simulink model "UAVbackstepping"  (Simulink 10.3)
settings: Solver=FixedStepAuto  StartTime=0.0  StopTime=100  FixedStep=0.01  RelTol=1e-3  EnableMultiTasking=on
settings Model: LogicAnalyzerSignalOrdering=b46eab1f-6d7b-46d5-ba77-869c9bcf8073,e372ee43-6b29-46b4-abe2-21db8a75f3db,54536452-6e4b-4c4e-8d4d-0328bb149ba5,ee120f98-b3af-4c2b-98e6-fd07fbf403a8,95f0ccf8-e806-4aca-b244-47a68f5b17c2,43173032-e17e-41b3-ae27-c107c89a8554,cd05f008-1193-4f09-83b2-320887a6bfed,77335dc1-2049-4d60-adff-c5cf65fb9f9c,2b0633ed-ee51-4564-bd40-7c1ecd56d7dd,dfe04f60-c018-4575-84ca-0f2bc48ccfdd,15828245-0370-4267-bd56-27ac584a7d3e,a94eabd6-13e1-4944-88ab-4db36129ad16,2589506c-7c8c-49ed-89a6-d105e2fe226b,cee16f5b-ea6a-452d-9ab2-cf488d9efbab,cfbac93e-1ce9-416b-a9d8-bf10efdf7acc,4b85f622-f658-405c-8f3b-f9afb204eecf,74d215f9-d3fc-487f-9be0-003869bd056c,b88364f3-47d2-4798-9ca3-2210a76b2151,992ed9bb-61c6-4816-9df8-a6a9b01ec379,fa3f50c4-9508-49a0-8b01-2ac87a115d50,443bea33-00d3-41d7-a326-92ebc5658bd2,b9b4d7ee-6fc8-43e3-85dd-aee403bc8ecc,493d881f-12cd-495e-8dbc-5128311b9c68,b5f602f6-6904-40bd-b13c-e30cee082fb3,ac9778e8-5991-4c7f-a0e3-96968d354415,7bf7420a-51df-410a-ad7d-640b8e127968,6783366a-253d-440d-8309-d3e37f712b7a,e3002545-8a11-46c6-8ec8-6cad10b13a30,8d9e8d02-f9c8-417c-9dde-eafb8a0edd13,386452ee-c7b4-48c3-9b3b-9b5c8c01b9d9,a3f579f7-78fa-4a39-bc72-402bae468470,1b92f911-6c45-4a57-9771-5ef78c83ee6e,46570d27-1e42-4fbc-a47b-5b7b35a38f8f,e5c679aa-f5c2-4db1-b0e0-4143dc9292e5,653c2844-e192-4241-9d80-46dbab4f59eb,a81b4801-5ad4-47ee-be3a-7b6b03c586a0,9c2d5a89-a715-4e09-b03f-f97d33dae6e2,bbe3c297-77a7-404c-8c78-a013d080af9d,25508a3f-0527-4920-9e54-841bdeffa537,04472a12-bcc6-4a52-8174-bab8d6a6428e,43579eec-1d9f-48b6-9500-b23169589754,13906945-f0a2-42b5-a059-d3263a4d8fea,5debfe0f-7549-4053-9490-66e9123c9aa5,ba1e7171-ac89-4725-b702-5e8a13beef21,88975c86-fcb6-4eb7-a3b3-cfbaa1f90a45,5938fb88-f0d0-465a-95d6-16780bbd5b65,12608a54-9dd1-42f3-95f2-303540ea6fbd,e0fdc368-fa77-4673-aa31-0c283bfe0d72,9baec6ec-eb92-460d-8517-da3730d3c5a9,b421fcc5-0c1c-4c89-ba38-a7c1f88a7f58,8eabe517-0bde-4a7e-9911-b56cb8fb40be,d2f80fa9-708b-426c-89bf-a5279d614744,4ff3bab7-3c7f-4ac4-b9a7-239084307073,16cb91f4-d8fb-4662-979f-86f54ca22852,694bc1bc-d9f8-4696-9709-c2a3c0b4c400,9b3c29cc-2abe-4d54-a9dd-6ec7aa243ded,9a8a996a-a39e-40af-b6f5-e33e96ef8062,4edc1bd5-7ef1-4e99-9f98-7b7c38d83df9,574ec7e1-1a45-4502-b5ca-a33a3001e453,54705b3a-a62a-42de-9894-18fee6dd9f2f,52cc81ea-ec29-4b3c-a7fa-d0b8a74c3977,40c87669-2e0a-4c05-aa3c-23dbde47ecaf,8d820c60-f138-442a-a396-16a173d0311b,099a5a67-d92d-4072-ac0a-dca54051a8b8,37013ffe-99d3-4146-a42e-9df11827c8f0  Creator=Administrator  LastModifiedBy=duolan  MultithreadedSim=on
settings DataIOCC: LimitDataPoints=on  SignalLoggingSaveFormat=Dataset
settings OptimizationCC: ExpressionDepthLimit=128
settings DebuggingCC: UnderspecifiedInitializationDetection=Simplified  MergeDetectMultiDrivingBlocksExec=error  SolverPrmCheckMsg=warning  FcnCallInpInsideContextMsg=error  StateNameClashWarn=none
settings GRTTargetCC: CombineOutputUpdateFcns=on  GRTInterface=off
settings ConfigComp: CovSFcnEnable=off

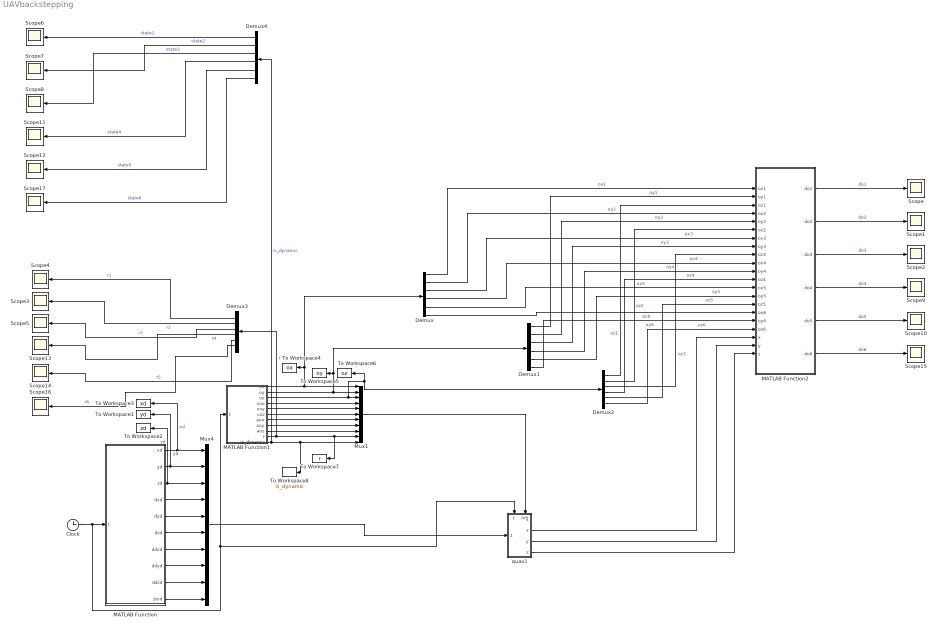
== system UAVbackstepping ==
  Clock : Clock
  Demux{,1..4} (5 alike) : Demux  Outputs=6
  MATLAB Function : MATLAB Function  TreatAsAtomicUnit=on
  MATLAB Function1 : MATLAB Function  TreatAsAtomicUnit=on
  MATLAB Function2 : MATLAB Function  TreatAsAtomicUnit=on
  Mux1 : Mux  Inputs=11
  Mux4 : Mux  Inputs=10
  Scope{,1..17} (18 alike) : Scope
  To Workspace1 : ToWorkspace  VariableName=yd  SampleTime=-1
  To Workspace2 : ToWorkspace  VariableName=zd  SampleTime=-1
  To Workspace3 : ToWorkspace  VariableName=xd  SampleTime=-1
  To Workspace4 : ToWorkspace  VariableName=ox  SampleTime=-1
  To Workspace5 : ToWorkspace  VariableName=oy  SampleTime=-1
  To Workspace6 : ToWorkspace  VariableName=oz  SampleTime=-1
  To Workspace7 : ToWorkspace  VariableName=r  SampleTime=-1
  To Workspace8 : ToWorkspace  VariableName=is_dynamic  SampleTime=-1
  quav1 : Subsystem
      settings: PortSchema="{\"entries\":[{\"content\":{\"sides\":[{\"content\":{\"connectorIds\":[\"In1\"]},\"type\":\"ConnectorPlacement.EquallySpacedRectSide\",\"uuid\":\"dcfd3588-1954-4120-b512-4285ff7746bb\"},{\"content\":{\"connectorIds\":[\"Out1\",\"Out2\",\"Out3\",\"Out4\"],\"side\":\"RIGHT\"},\"type\":\"ConnectorPlacement.EquallySpacedRectSide\",\"uuid\":\"6db42291-2fd7-4549-90c1-3af3d88c1f44\"},{\"content\":{\"connectorIds\":[\"In2\",\"In3\"],\"side\":\"TOP\"},\"type\":\"ConnectorPlacement.EquallySpacedRectSide\",\"uuid\":\"9b3b6533-6a28-4d06-948b-5572cd3b642f\"}]},\"type\":\"ConnectorPlacement.EquallySpacedConnector\",\"uuid\":\"66a38cae-fd35-47b9-aceb-4f0f598ddd12\"}],\"packageUris\":[\"http://schema.mathworks.com/mf0/Connector/R2020b\"],\"version\":\"1.0\"}"
  wires:
  MATLAB Function/2(yd) -> To Workspace1/1, Mux4/2  "yd"
  MATLAB Function/3(zd) -> Mux4/3, To Workspace2/1  "zd"
  MATLAB Function/1(xd) -> To Workspace3/1, Mux4/1  "xd"
  MATLAB Function/4(dxd) -> Mux4/4
  MATLAB Function/5(dyd) -> Mux4/5
  MATLAB Function/6(dzd) -> Mux4/6
  MATLAB Function/7(ddxd) -> Mux4/7
  MATLAB Function/8(ddyd) -> Mux4/8
  MATLAB Function/9(ddzd) -> Mux4/9
  MATLAB Function/10(psid) -> Mux4/10
  Mux4/1 -> quav1/1(In1)
  Clock/1 -> quav1/2(t), MATLAB Function1/1(t), MATLAB Function/1(t)
  MATLAB Function1/1(ox) -> Mux1/1, Demux/1, To Workspace4/1
  MATLAB Function1/2(oy) -> Mux1/2, Demux1/1, To Workspace5/1
  MATLAB Function1/3(oz) -> Mux1/3, To Workspace6/1, Demux2/1
  Mux1/1 -> quav1/3(In5)
  MATLAB Function1/4(vox) -> Mux1/4
  MATLAB Function1/5(voy) -> Mux1/5
  MATLAB Function1/6(voz) -> Mux1/6
  MATLAB Function1/7(aox) -> Mux1/7
  MATLAB Function1/8(aoy) -> Mux1/8
  MATLAB Function1/9(aoz) -> Mux1/9
  MATLAB Function1/10(r) -> Demux3/1, To Workspace7/1, Mux1/10  "r"
  MATLAB Function1/11(is_dynamic) -> To Workspace8/1, Mux1/11, Demux4/1  "is_dynamic"
  MATLAB Function2/1(do1) -> Scope/1  "do1"
  MATLAB Function2/2(do2) -> Scope1/1  "do2"
  MATLAB Function2/3(do3) -> Scope2/1  "do3"
  quav1/2(x) -> MATLAB Function2/19(x)
  quav1/3(y) -> MATLAB Function2/20(y)
  quav1/4(z) -> MATLAB Function2/21(z)
  Demux3/1 -> Scope4/1  "r1"
  Demux3/2 -> Scope3/1  "r2"
  Demux3/3 -> Scope5/1  "r3"
  Demux4/1 -> Scope6/1  "state1"
  Demux4/2 -> Scope7/1  "state2"
  Demux4/3 -> Scope8/1  "state3"
  Demux/1 -> MATLAB Function2/1(ox1)  "ox1"
  Demux1/1 -> MATLAB Function2/2(oy1)  "oy1"
  Demux2/1 -> MATLAB Function2/3(oz1)  "oz1"
  Demux/2 -> MATLAB Function2/4(ox2)  "ox2"
  Demux1/2 -> MATLAB Function2/5(oy2)  "oy2"
  Demux2/2 -> MATLAB Function2/6(oz2)  "oz2"
  Demux/3 -> MATLAB Function2/7(ox3)  "ox3"
  Demux1/3 -> MATLAB Function2/8(oy3)  "oy3"
  Demux2/3 -> MATLAB Function2/9(oz3)  "oz3"
  Demux/4 -> MATLAB Function2/10(ox4)  "ox4"
  Demux1/4 -> MATLAB Function2/11(oy4)  "oy4"
  Demux/5 -> MATLAB Function2/13(ox5)  "ox5"
  Demux1/5 -> MATLAB Function2/14(oy5)  "oy5"
  Demux2/5 -> MATLAB Function2/15(oz5)  "oz5"
  MATLAB Function2/4(do4) -> Scope9/1  "do4"
  MATLAB Function2/5(do5) -> Scope10/1  "do5"
  Demux2/4 -> MATLAB Function2/12(oz4)  "oz4"
  Demux4/4 -> Scope11/1  "state4"
  Demux4/5 -> Scope12/1  "state5"
  Demux3/4 -> Scope13/1  "r4"
  Demux3/5 -> Scope14/1  "r5"
  Demux/6 -> MATLAB Function2/16(ox6)  "ox6"
  Demux1/6 -> MATLAB Function2/17(oy6)  "oy6"
  Demux2/6 -> MATLAB Function2/18(oz6)  "oz6"
  MATLAB Function2/6(do6) -> Scope15/1  "do6"
  Demux3/6 -> Scope16/1  "r6"
  Demux4/6 -> Scope17/1  "state6"

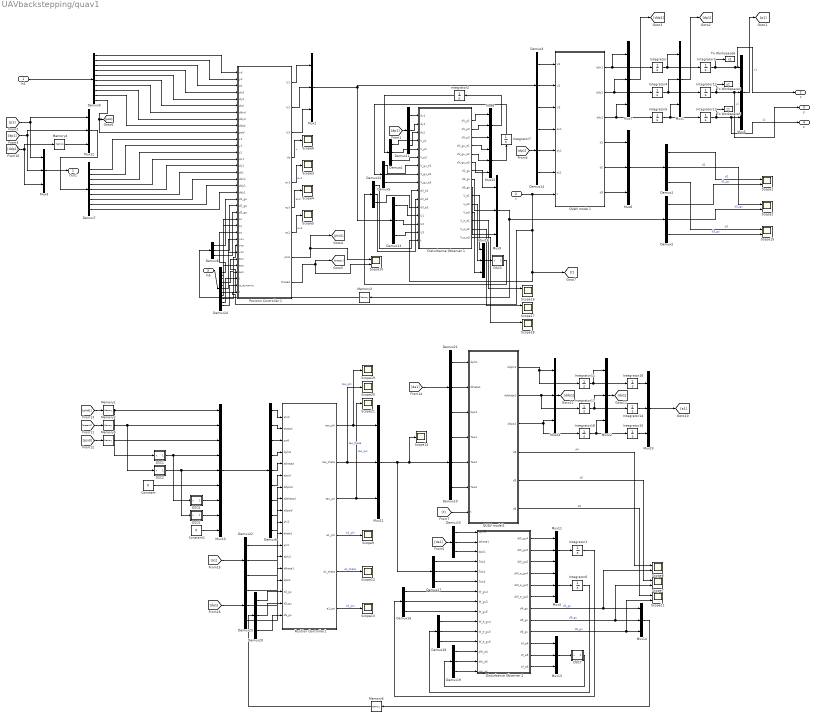
== system UAVbackstepping/quav1 ==
  In1 : Inport
  t : Inport  Port=2
  In5 : Inport  Port=3
  Constant : Constant  Value=0
  Constant1 : Constant  Value=0
  DSC1 : Subsystem
  DSC2 : Subsystem
  DSC3 : Subsystem
  DSC4 : Subsystem
  DSC5 : Subsystem
  DSC7 : Subsystem
  Demux{1..5,8,10..23} (20 alike) : Demux  Outputs=3
  Demux24 : Demux  Outputs=11
  Demux6 : Demux  Outputs=9
  Demux7 : Demux  Outputs=9
  Demux9 : Demux  Outputs=10
  Disturbance Observer 1 : MATLAB Function  TreatAsAtomicUnit=on
  Disturbance Observer 2 : MATLAB Function  TreatAsAtomicUnit=on
  Integrator{,1..2,4..7,11..18} (15 alike) : Integrator
  Integrator3 : Integrator  InitialCondition=1
  Memory{1..4,6} (5 alike) : Memory
  Memory5 : Memory  InitialCondition=pi/3
  Mux{1..9,11..16,21..24} (19 alike) : Mux  Inputs=3
  Mux10 : Mux  Inputs=9
  Position Controller 1 : MATLAB Function  TreatAsAtomicUnit=on
  Position Controller1 : MATLAB Function  TreatAsAtomicUnit=on
  QUAV mode 1 : MATLAB Function  TreatAsAtomicUnit=on
  QUAV model1 : MATLAB Function  TreatAsAtomicUnit=on
  Scope{1..2,7..8,10..11,15..18} (10 alike) : Scope  NumInputPorts=2
  Scope{3..6,9,12..14,19..21} (11 alike) : Scope
  To Workspace4 : ToWorkspace  VariableName=y1  SampleTime=-1
  To Workspace5 : ToWorkspace  VariableName=z1  SampleTime=-1
  To Workspace6 : ToWorkspace  VariableName=x1  SampleTime=-1
  Out1 : Outport
  x : Outport  Port=2
  y : Outport  Port=3
  z : Outport  Port=4
  wires:
  Demux7/5 -> Position Controller 1/15(dy1)
  Position Controller 1/2(U2) -> Mux1/2
  QUAV mode 1/1(ddx1) -> Mux7/1, Integrator/1
  QUAV mode 1/3(ddz1) -> Mux7/3, Integrator5/1
  Disturbance Observer 1/2(dV_p2) -> Mux8/2
  Demux7/7 -> Position Controller 1/17(ddx1)
  Demux8/2 -> Position Controller 1/21(d2_gu)
  Integrator13/1 -> z/1, Mux5/3, To Workspace5/1  "z1"
  Demux7/3 -> Position Controller 1/13(z1)
  Disturbance Observer 1/9(d3_gu) -> Mux9/3
  Demux11/1 -> Disturbance Observer 1/1(dx1)
  Demux9/8 -> Position Controller 1/8(ddyd)
  Integrator4/1 -> Mux2/2, Integrator12/1
  Mux1/1 -> Demux3/1, Demux13/1
  Demux7/6 -> Position Controller 1/16(dz1)
  Demux9/3 -> Position Controller 1/3(zd)
  Demux9/10 -> [psid], Position Controller 1/10(psid)
  QUAV mode 1/5(d2) -> Mux6/2
  [dp1] -> Demux14/1
  Memory3/1 -> Demux8/1
  Demux3/3 -> QUAV mode 1/3(U3)
  Mux2/1 -> [dp1]
  Demux7/8 -> Position Controller 1/18(ddy1)
  Demux3/2 -> QUAV mode 1/2(U2)
  Demux7/9 -> Position Controller 1/19(ddz1)
  Demux14/3 -> QUAV mode 1/6(dz1)
  QUAV mode 1/2(ddy1) -> Mux7/2, Integrator4/1
  Demux9/6 -> Position Controller 1/6(dzd)
  Demux14/2 -> QUAV mode 1/5(dy1)
  [ddp1] -> Mux3/3, Memory4/1
  Position Controller 1/1(U1) -> Mux1/1
  Demux9/7 -> Position Controller 1/7(ddxd)
  Integrator5/1 -> Mux2/3, Integrator13/1
  Integrator/1 -> Mux2/1, Integrator3/1
  Demux3/1 -> QUAV mode 1/1(U1)
  QUAV mode 1/6(d3) -> Mux6/3
  Demux9/4 -> Position Controller 1/4(dxd)
  Position Controller 1/4(Up) -> Scope6/1  "u"
  Memory4/1 -> Mux12/3
  Demux13/1 -> Disturbance Observer 1/13(U1)
  Demux7/4 -> Position Controller 1/14(dx1)
  Demux11/2 -> Disturbance Observer 1/2(dy1)
  Mux6/1 -> Demux1/1
  Mux5/1 -> [p1]
  Demux13/3 -> Disturbance Observer 1/15(U3)
  Disturbance Observer 1/7(d1_gu) -> Mux9/1
  Disturbance Observer 1/8(d2_gu) -> Mux9/2
  Demux14/1 -> QUAV mode 1/4(dx1)
  Mux7/1 -> [ddp1]
  QUAV mode 1/4(d1) -> Mux6/1
  Demux11/3 -> Disturbance Observer 1/3(dz1)
  Position Controller 1/3(U3) -> Mux1/3
  Demux7/1 -> Position Controller 1/11(x1)
  Disturbance Observer 1/3(dV_p3) -> Mux8/3
  [dp1] -> Demux11/1
  Position Controller 1/6(ey1) -> Scope4/1  "ex2"
  Demux7/2 -> Position Controller 1/12(y1)
  Demux13/2 -> Disturbance Observer 1/14(U2)
  Disturbance Observer 1/1(dV_p1) -> Mux8/1
  Mux12/1 -> Demux7/1
  Position Controller 1/5(ex1) -> Scope3/1  "ex1"
  Integrator3/1 -> x/1, Mux5/1, To Workspace6/1  "x1"
  Demux8/3 -> Position Controller 1/22(d3_gu)
  Demux9/5 -> Position Controller 1/5(dyd)
  [dp1] -> Mux3/2, Mux12/2
  Position Controller 1/7(ez1) -> Scope5/1  "ex3"
  [p1] -> Mux3/1, Mux12/1
  Demux9/1 -> Position Controller 1/1(xd)
  Demux8/1 -> Position Controller 1/20(d1_gu)
  Demux9/2 -> Position Controller 1/2(yd)
  Demux9/9 -> Position Controller 1/9(ddzd)
  Integrator12/1 -> y/1, Mux5/2, To Workspace4/1  "y1"
  Mux9/1 -> Memory3/1, Demux2/1
  Mux8/1 -> Integrator2/1
  In1/1 -> Demux9/1
  Mux3/1 -> Out1/1
  t/1 -> Position Controller 1/34(t), Disturbance Observer 1/16(t), [t], QUAV mode 1/7(t)
  Position Controller 1/8(phid) -> [phid1], Scope10/1
  Position Controller 1/9(thetad) -> Scope10/2, [thetad1]
  QUAV model1/1(ddphi1) -> Integrator11/1, Mux24/1
  Mux22/1 -> [da1]
  Mux23/1 -> [a1]
  Demux6/7 -> Position Controller1/7(ddphid)
  Integrator14/1 -> Mux23/2
  [phid1] -> Memory1/1
  Demux23/1 -> Position Controller1/13(dphi1)
  Demux6/5 -> Position Controller1/5(dthetad)
  Position Controller1/6(e1_psi) -> Scope13/1  "e1_psi"
  Constant/1 -> Mux10/6
  Position Controller1/1(tao_phi) -> Scope19/1, Mux21/1  "tao_phi"
  Demux22/1 -> Position Controller1/10(phi1)
  Demux22/2 -> Position Controller1/11(theta1)
  DSC5/1(dx) -> Mux10/8
  Demux23/3 -> Position Controller1/15(dpsi1)
  Demux10/2 -> QUAV model1/5(Tao2)
  Demux6/8 -> Position Controller1/8(ddthetad)
  [thetad1] -> Memory2/1
  Position Controller1/4(e1_phi) -> Scope9/1  "e1_phi"
  Position Controller1/5(e1_theta) -> Scope12/1  "e1_theta"
  Demux10/1 -> QUAV model1/4(Tao1)
  [psid] -> Memory5/1
  Demux21/3 -> QUAV model1/3(dpsi1)
  DSC1/1(dx) -> DSC4/1(x), Mux10/4
  Demux21/1 -> QUAV model1/1(dphi1)
  Constant1/1 -> Mux10/9
  [da1] -> Demux23/1
  Demux21/2 -> QUAV model1/2(dtheta1)
  Demux23/2 -> Position Controller1/14(dtheta1)
  [da1] -> Demux21/1
  Integrator15/1 -> Mux23/3
  DSC2/1(dx) -> DSC5/1(x), Mux10/5
  Integrator18/1 -> Mux22/3, Integrator15/1
  QUAV model1/3(ddpsi1) -> Integrator18/1, Mux24/3
  Demux6/4 -> Position Controller1/4(dphid)
  Integrator11/1 -> Mux22/1, Integrator16/1
  Integrator17/1 -> Mux22/2, Integrator14/1
  Integrator16/1 -> Mux23/1
  Position Controller1/2(tao_theta) -> Scope20/1, Mux21/2  "tao_theta"
  Demux6/6 -> Position Controller1/6(dpsid)
  Position Controller1/3(tao_psi) -> Scope21/1, Mux21/3  "tao_psi"
  Mux10/1 -> Demux6/1
  [a1] -> Demux22/1
  Demux22/3 -> Position Controller1/12(psi1)
  Demux10/3 -> QUAV model1/6(Tao3)
  Demux6/9 -> Position Controller1/9(ddpsid)
  QUAV model1/2(ddtheta1) -> Integrator17/1, Mux24/2
  Mux21/1 -> Demux17/1, Scope14/1, Demux10/1
  Demux6/1 -> Position Controller1/1(phid)
  Demux6/3 -> Position Controller1/3(psid)
  DSC4/1(dx) -> Mux10/7
  Mux24/1 -> [dda1]
  Demux6/2 -> Position Controller1/2(thetad)
  Demux15/1 -> Disturbance Observer 2/1(dphi1)
  Demux15/2 -> Disturbance Observer 2/2(dtheta1)
  Demux15/3 -> Disturbance Observer 2/3(dpsi1)
  Disturbance Observer 2/1(dW_gu4) -> Mux11/1
  Disturbance Observer 2/2(dW_gu5) -> Mux11/2
  Disturbance Observer 2/3(dW_gu6) -> Mux11/3
  Mux11/1 -> Integrator1/1
  [da1] -> Demux15/1
  [t] -> QUAV model1/7(t)
  QUAV model1/4(d4) -> Scope8/1  "d4"
  QUAV model1/5(d5) -> Scope7/1  "d5"
  QUAV model1/6(d6) -> Scope11/1  "d6"
  Demux16/1 -> Disturbance Observer 2/7(W_gu4)
  Demux16/2 -> Disturbance Observer 2/8(W_gu5)
  Demux16/3 -> Disturbance Observer 2/9(W_gu6)
  Integrator1/1 -> Demux16/1
  Demux17/1 -> Disturbance Observer 2/4(Tao1)
  Demux17/2 -> Disturbance Observer 2/5(Tao2)
  Demux17/3 -> Disturbance Observer 2/6(Tao3)
  Disturbance Observer 2/7(d4_gu) -> Mux14/1, Scope8/2  "d4_gu"
  Disturbance Observer 2/8(d5_gu) -> Mux14/2, Scope7/2  "d5_gu"
  Disturbance Observer 2/9(d6_gu) -> Mux14/3, Scope11/2  "d6_gu"
  Disturbance Observer 2/5(dW_e_gu5) -> Mux4/2
  Disturbance Observer 2/4(dW_e_gu4) -> Mux4/1
  Mux4/1 -> Integrator6/1
  Disturbance Observer 2/6(dW_e_gu6) -> Mux4/3
  Demux18/1 -> Disturbance Observer 2/10(W_e_gu4)
  Demux18/2 -> Disturbance Observer 2/11(W_e_gu5)
  Demux18/3 -> Disturbance Observer 2/12(W_e_gu6)
  Integrator6/1 -> Demux18/1
  Disturbance Observer 2/10(W_e4) -> Mux13/1
  Disturbance Observer 2/11(W_e5) -> Mux13/2
  Disturbance Observer 2/12(W_e6) -> Mux13/3
  Mux13/1 -> DSC7/1(x)
  Demux19/1 -> Disturbance Observer 2/13(dW_e4)
  Demux19/2 -> Disturbance Observer 2/14(dW_e5)
  Demux19/3 -> Disturbance Observer 2/15(dW_e6)
  DSC7/1(dx) -> Demux19/1
  Mux14/1 -> Memory6/1
  Demux20/1 -> Position Controller1/16(d4_gu)
  Demux20/2 -> Position Controller1/17(d5_gu)
  Demux20/3 -> Position Controller1/18(d6_gu)
  Memory6/1 -> Demux20/1
  Memory1/1 -> DSC1/1(x), Mux10/1
  Memory2/1 -> DSC2/1(x), Mux10/2
  Memory5/1 -> Mux10/3
  In5/1 -> Demux24/1
  Demux24/1 -> Position Controller 1/23(ox)
  Demux24/2 -> Position Controller 1/24(oy)
  Demux24/3 -> Position Controller 1/25(oz)
  Demux24/4 -> Position Controller 1/26(vox)
  Demux24/5 -> Position Controller 1/27(voy)
  Demux24/6 -> Position Controller 1/28(voz)
  Demux24/7 -> Position Controller 1/29(aox)
  Demux24/8 -> Position Controller 1/30(aoy)
  Demux24/9 -> Position Controller 1/31(aoz)
  Demux24/10 -> Position Controller 1/32(r)
  Demux24/11 -> Position Controller 1/33(is_dynamic)
  Integrator2/1 -> Demux4/1
  Demux4/1 -> Disturbance Observer 1/4(V_p1)
  Demux4/2 -> Disturbance Observer 1/5(V_p2)
  Demux4/3 -> Disturbance Observer 1/6(V_p3)
  Disturbance Observer 1/4(dV_gu_e1) -> Mux15/1
  Disturbance Observer 1/5(dV_gu_e2) -> Mux15/2
  Disturbance Observer 1/6(dV_gu_e3) -> Mux15/3
  Mux15/1 -> Integrator7/1
  Integrator7/1 -> Demux5/1
  Demux5/1 -> Disturbance Observer 1/7(V_gu_e1)
  Demux5/2 -> Disturbance Observer 1/8(V_gu_e2)
  Demux5/3 -> Disturbance Observer 1/9(V_gu_e3)
  Disturbance Observer 1/10(V_e1) -> Mux16/1
  Disturbance Observer 1/11(V_e2) -> Mux16/2
  Disturbance Observer 1/12(V_e3) -> Mux16/3
  Mux16/1 -> DSC3/1(x)
  DSC3/1(dx) -> Demux12/1
  Demux12/1 -> Disturbance Observer 1/10(dV_e1)
  Demux12/2 -> Disturbance Observer 1/11(dV_e2)
  Demux12/3 -> Disturbance Observer 1/12(dV_e3)
  Demux1/1 -> Scope1/1  "d1"
  Demux2/1 -> Scope1/2  "d1_gu"
  Demux1/2 -> Scope2/1  "d2"
  Demux2/2 -> Scope2/2  "d2_gu"
  Demux1/3 -> Scope15/1  "d3"
  Demux2/3 -> Scope15/2  "d3_gu"
  Disturbance Observer 1/13(V_e_e1) -> Scope16/1
  Disturbance Observer 1/14(V_e_e2) -> Scope17/1
  Disturbance Observer 1/15(V_e_e3) -> Scope18/1

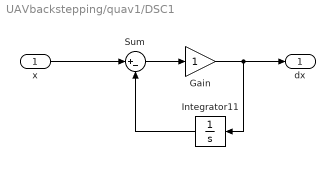
== system UAVbackstepping/quav1/DSC1 ==
  x : Inport
  Gain : Gain
  Integrator11 : Integrator
  Sum : Sum  Inputs=|+-
  dx : Outport
  wires:
  Sum/1 -> Gain/1
  x/1 -> Sum/1
  Integrator11/1 -> Sum/2
  Gain/1 -> Integrator11/1, dx/1

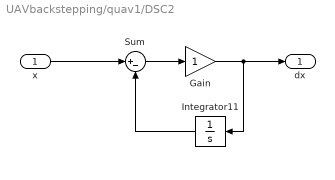
== system UAVbackstepping/quav1/DSC2 ==
  x : Inport
  Gain : Gain
  Integrator11 : Integrator
  Sum : Sum  Inputs=|+-
  dx : Outport
  wires:
  Sum/1 -> Gain/1
  x/1 -> Sum/1
  Integrator11/1 -> Sum/2
  Gain/1 -> Integrator11/1, dx/1

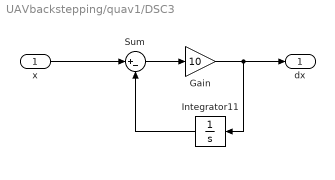
== system UAVbackstepping/quav1/DSC3 ==
  x : Inport
  Gain : Gain  Gain=10
  Integrator11 : Integrator
  Sum : Sum  Inputs=|+-
  dx : Outport
  wires:
  Sum/1 -> Gain/1
  x/1 -> Sum/1
  Integrator11/1 -> Sum/2
  Gain/1 -> Integrator11/1, dx/1

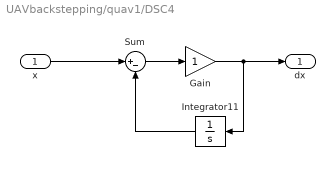
== system UAVbackstepping/quav1/DSC4 ==
  x : Inport
  Gain : Gain
  Integrator11 : Integrator
  Sum : Sum  Inputs=|+-
  dx : Outport
  wires:
  Sum/1 -> Gain/1
  x/1 -> Sum/1
  Integrator11/1 -> Sum/2
  Gain/1 -> Integrator11/1, dx/1

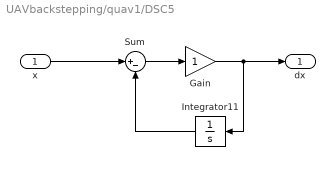
== system UAVbackstepping/quav1/DSC5 ==
  x : Inport
  Gain : Gain
  Integrator11 : Integrator
  Sum : Sum  Inputs=|+-
  dx : Outport
  wires:
  Sum/1 -> Gain/1
  x/1 -> Sum/1
  Integrator11/1 -> Sum/2
  Gain/1 -> Integrator11/1, dx/1

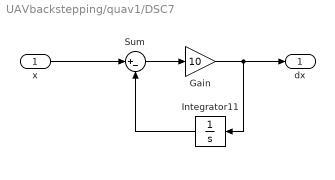
== system UAVbackstepping/quav1/DSC7 ==
  x : Inport
  Gain : Gain  Gain=10
  Integrator11 : Integrator
  Sum : Sum  Inputs=|+-
  dx : Outport
  wires:
  Sum/1 -> Gain/1
  x/1 -> Sum/1
  Integrator11/1 -> Sum/2
  Gain/1 -> Integrator11/1, dx/1

== matlab function quav1/Position Controller 1 ==
  data: xd input double; U1 output double; yd input double; zd input double; dxd input double; dyd input double; dzd input double; ddxd input double; ddyd input double; ddzd input double; psid input double; x1 input double; y1 input double; z1 input double; dx1 input double; dy1 input double; dz1 input double; ddx1 input double; ddy1 input double; ddz1 input double; U2 output double; U3 output double; Up output double; ex1 output double; ey1 output double; ez1 output double; d1_gu input double; d2_gu input double; d3_gu input double; phid output double; thetad output double; ox input double; oy input double; oz input double; vox input double; voy input double; voz input double; aox input double; aoy input double; aoz input double; r input double; is_dynamic input double; t input double
function [U1,U2,U3,Up,ex1,ey1,ez1,phid,thetad] = fcn(xd,yd,zd,dxd,dyd,dzd,ddxd,ddyd,ddzd,psid,x1,y1,z1,dx1,dy1,dz1,ddx1,ddy1,ddz1,d1_gu,d2_gu,d3_gu,ox,oy,oz,vox,voy,voz,aox,aoy,aoz,r,is_dynamic,t)

%postion parameter
K1=0.1;
K2=0.1;
K3=0.1;
m=2;
g=9.81;
es=0.01;


% error
ex1=x1-xd;
dex1=dx1-dxd;
ey1=y1-yd;
dey1=dy1-dyd;
ez1=z1-zd;
dez1=dz1-dzd;


% nominal control
es=0.01;
kex11=0.65;kex12=7/9;kex13=(2-kex12)*es^(kex12-1);kex14=(kex12-1)*es^(kex12-2);b1=0.65;
key11=0.5;key12=7/9;key13=(2-key12)*es^(key12-1);key14=(key12-1)*es^(key12-2);b2=0.5;
kez11=2.5;kez12=7/9;kez13=(2-kez12)*es^(kez12-1);kez14=(kez12-1)*es^(kez12-2);b3=2.5;

if abs(ex1)>es
    Lx1=kex11*((abs(ex1))^kex12)*sign(ex1);
else
    Lx1=kex13*ex1+kex14*ex1*ex1*sign(ex1);
end
if abs(ey1)>es
    Ly1=key11*((abs(ey1))^key12)*sign(ey1);
else
    Ly1=key13*ey1+key14*ey1*ey1*sign(ey1);
end
if abs(ez1)>es
    Lz1=kez11*((abs(ez1))^(kez12))*sign(ez1);
else
    Lz1=kez13*ez1+key14*ez1*ez1*sign(ez1);
end
sx1=dex1+b1*ex1+Lx1;
sy1=dey1+b2*ey1+Ly1;
sz1=dez1+b3*ez1+Lz1;

if abs(ex1)>es
    dLx1=kex11*kex12*((abs(ex1))^(kex12-1))*dex1;
else 
    dLx1=kex13*dex1+2*kex14*ex1*dex1*sign(ex1);
end
if abs(ey1)>es
    dLy1=key11*key12*((abs(ey1))^(key12-1))*dey1;
else
    dLy1=key13*dey1+2*key14*ey1*dey1*sign(ey1);
end
if abs(ez1)>es
    dLz1=kez11*kez12*((abs(ez1))^(kez12-1))*dez1;
else
    dLz1=kez13*dez1+2*kez14*ez1*dez1*sign(ez1);
end

U1=K1*dx1/m-d1_gu+ddxd-b1*dex1-dLx1-5*sx1-5*((abs(sx1))^(5/7))*sign(sx1);
U2=K2*dy1/m-d2_gu+ddyd-b2*dey1-dLy1-1.5*sy1-1.5*((abs(sy1))^(5/7))*sign(sy1);
U3=K3*dz1/m-d3_gu+g+ddzd-b3*dez1-dLz1-1.5*sz1-1.5*((abs(sz1))^(5/7))*sign(sz1);




%control barrier function
k1 = 4; k2 = 4;

num_obs = length(ox);  
A = zeros(num_obs, 3); 
b = zeros(num_obs, 1);

for i = 1:num_obs
    oxi = ox(i);
    oyi = oy(i);
    ozi = oz(i);
    voxi = vox(i);
    voyi = voy(i);
    vozi = voz(i);
    aoxi = aox(i);
    aoyi = aoy(i);
    aozi = aoz(i);
    ri  = r(i);
    
    % 
    h = (x1 - oxi)^2 + (y1 - oyi)^2 + (z1 - ozi)^2 - (ri+0.2)^2;
    dh = 2*(x1 - oxi)*(-voxi)+2*(x1 - oxi)*dx1 +2*(y1 - oyi)*(-voyi)+ 2*(y1 - oyi)*dy1 + 2*(z1 - ozi)*(-vozi)+2*(z1 - ozi)*dz1;
    dh1=2*(x1 - oxi)*dx1+ 2*(y1 - oyi)*dy1+2*(z1 - ozi)*dz1;
    % 
    A(i, :) = [-2*(x1 - oxi), -2*(y1 - oyi), -2*(z1 - ozi)];


    b(i) = 2*(x1 - oxi)*(-K1*dx1/m+d1_gu )-abs(2*(x1 - oxi))*2.5+ 2*(dx1^2)+2*(voxi^2)-4*voxi*dx1-2*(x1 - oxi)*aoxi+ ...
           2*(y1 - oyi)*(-K2*dy1/m+d2_gu )+ 2*(dy1^2)+2*(voyi^2)-4*voyi*dy1-2*(y1 - oyi)*aoyi +...
           2*(z1 - ozi)*(-K3*dz1/m - g+d3_gu)+ 2*(dz1^2)+2*(vozi^2)-4*vozi*dz1-2*(z1 - ozi)*aozi+ ...
           k1*h + k2*dh;
end


% QP
u_tsmc = [U1, U2, U3];
u0 = [0, 0, 0]; 
H = eye(3); 
f = -u_tsmc;
options = optimoptions('quadprog', 'Algorithm', 'active-set', 'Display', 'none');
[u_opt, ~, exitflag] = quadprog(H, f, A, b, [], [], [], [], u0, options);

if exitflag > 0
    U1 = u_opt(1);
    U2 = u_opt(2);
    U3 = u_opt(3);
else
    U1 = u_tsmc(1);
    U2 = u_tsmc(2);
    U3 = u_tsmc(3);
end




%optimal control
Up=sqrt(U1^2+U2^2+U3^2);


% desired att 
Pphid=(sin(psid)*U1-cos(psid)*U2)/Up;
if abs(Pphid)>sin(pi/3)
    if Pphid>0
        phid=pi/3;
    else
        phid=-pi/3;
    end
else 
    phid=asin(Pphid);
end

Pthetad=(cos(psid)*U1+sin(psid)*U2)/U3;
if abs(Pthetad)>sin(pi/3)
    if Pthetad>0
        thetad=pi/3;
    else 
        thetad=-pi/3;
    end
else 
    thetad=atan(Pthetad);
end

== matlab function MATLAB Function ==
  data: t input double; xd output double; yd output double; zd output double; dxd output double; dyd output double; dzd output double; ddxd output double; ddyd output double; ddzd output double; psid output double
function [xd,yd,zd,dxd,dyd,dzd,ddxd,ddyd,ddzd,psid] = fcn(t)

psid=pi/3;
v = 0.5;  

% 
xd = v * t;
yd = v * t;
zd = 1;

% 
dxd = v;
dyd = v;
dzd = 0;

% 
ddxd = 0;
ddyd = 0;
ddzd = 0;

end

== matlab function quav1/Disturbance Observer 1 ==
  data: dx1 input double; dy1 input double; dz1 input double; V_p1 input double; dV_p1 output double; V_p2 input double; V_p3 input double; V_gu_e1 input double; V_gu_e2 input double; V_gu_e3 input double; dV_e1 input double; dV_e2 input double; dV_e3 input double; U1 input double; U2 input double; U3 input double; dV_p2 output double; dV_p3 output double; dV_gu_e1 output double; dV_gu_e2 output double; dV_gu_e3 output double; d1_gu output double; d2_gu output double; d3_gu output double; V_e1 output double; V_e2 output double; V_e3 output double; t input double; V_e_e1 output double; V_e_e2 output double; V_e_e3 output double
function [dV_p1,dV_p2,dV_p3,dV_gu_e1,dV_gu_e2,dV_gu_e3,d1_gu,d2_gu,d3_gu,V_e1,V_e2,V_e3,V_e_e1,V_e_e2,V_e_e3] = fcn(dx1,dy1,dz1,V_p1,V_p2,V_p3,V_gu_e1,V_gu_e2,V_gu_e3,dV_e1,dV_e2,dV_e3,U1,U2,U3,t)


%parameter po
K1=0.1;
K2=0.1;
K3=0.1;
m=2;
g=9.81;

%parameter DOB
k1=1;
k2=1;
k3=1;
k4=0.1;
k5=3/5;
k6=0.1;
k7=7/5;
k8=0.1;

%
V_e1=dx1-V_p1;
V_e2=dy1-V_p2;
V_e3=dz1-V_p3;

dV_p1=U1-K1*dx1/m+k1*V_e1;
dV_p2=U2-K2*dy1/m+k2*V_e2;
dV_p3=U3-K3*dz1/m-g+k3*V_e3;

V_e_e1=V_gu_e1-V_e1;
V_e_e2=V_gu_e2-V_e2;
V_e_e3=V_gu_e3-V_e3;

dV_gu_e1=dV_e1-k4*(sign(V_e_e1)*abs(V_e_e1)^k5)-k6*(sign(V_e_e1)*abs(V_e_e1)^k7)-k8*V_e_e1;
dV_gu_e2=dV_e2-k4*(sign(V_e_e2)*abs(V_e_e2)^k5)-k6*(sign(V_e_e2)*abs(V_e_e2)^k7)-k8*V_e_e2;
dV_gu_e3=dV_e3-k4*(sign(V_e_e3)*abs(V_e_e3)^k5)-k6*(sign(V_e_e3)*abs(V_e_e3)^k7)-k8*V_e_e3;

d1_gu=k1*V_gu_e1+dV_e1;
d2_gu=k2*V_gu_e2+dV_e2;
d3_gu=k3*V_gu_e3+dV_e3;

== matlab function quav1/QUAV mode 1 ==
  data: U1 input double; U2 input double; U3 input double; dx1 input double; dy1 input double; dz1 input double; ddx1 output double; ddy1 output double; ddz1 output double; d1 output double; d2 output double; d3 output double; t input double
function [ddx1,ddy1,ddz1,d1,d2,d3] = fcn(U1,U2,U3,dx1,dy1,dz1,t)


%parameter po
K1=0.1;K2=0.1;K3=0.1;m=2;



%disturbance
d1=0.5*sin(t)+0.8*cos(2*t);
d2=1.1*sin(t)+0.4*cos(3*t);
d3=0.6*sin(2*t)+0.8*cos(t);



ddx1=U1-K1*dx1/m+d1;
ddy1=U2-K2*dy1/m+d2;
ddz1=U3-9.81-K3*dz1/m+d3;

== matlab function MATLAB Function2 ==
  data: ox1 input double; do1 output double; do2 output double; do3 output double; oy1 input double; oz1 input double; ox2 input double; oy2 input double; oz2 input double; ox3 input double; oy3 input double; oz3 input double; ox4 input double; oy4 input double; oz4 input double; ox5 input double; oy5 input double; oz5 input double; ox6 input double; oy6 input double; oz6 input double; x input double; y input double; z input double; do4 output double; do5 output double; do6 output double
function [do1,do2,do3,do4,do5,do6] = fcn(ox1,oy1,oz1,ox2,oy2,oz2,ox3,oy3,oz3,ox4,oy4,oz4,ox5,oy5,oz5,ox6,oy6,oz6,x,y,z)

do1=sqrt((ox1-x)^2+(oy1-y)^2+(oz1-z)^2);
do2=sqrt((ox2-x)^2+(oy2-y)^2+(oz2-z)^2);
do3=sqrt((ox3-x)^2+(oy3-y)^2+(oz3-z)^2);
do4=sqrt((ox4-x)^2+(oy4-y)^2+(oz4-z)^2);
do5=sqrt((ox5-x)^2+(oy5-y)^2+(oz5-z)^2);
do6=sqrt((ox6-x)^2+(oy6-y)^2+(oz6-z)^2);





end

== matlab function quav1/Position Controller1 ==
  data: phid input double; tao_phi output double; tao_theta output double; tao_psi output double; e1_phi output double; e1_theta output double; e1_psi output double; thetad input double; psid input double; dphid input double; dthetad input double; dpsid input double; ddphid input double; ddthetad input double; ddpsid input double; phi1 input double; theta1 input double; psi1 input double; dphi1 input double; dtheta1 input double; dpsi1 input double; d4_gu input double; d5_gu input double; d6_gu input double
function [tao_phi,tao_theta,tao_psi,e1_phi,e1_theta,e1_psi] = fcn(phid,thetad,psid,dphid,dthetad,dpsid,ddphid,ddthetad,ddpsid,phi1,theta1,psi1,dphi1,dtheta1,dpsi1,d4_gu,d5_gu,d6_gu)

%parameter att
K4=0.1;K5=0.1;K6=0.1;
Ix=1.2416;Iy=1.2416;Iz=2.4832;l=0.2;


%error
e1_phi=phi1-phid;
de1_phi=dphi1-dphid;
e1_theta=theta1-thetad;
de1_theta=dtheta1-dthetad;
e1_psi=psi1-psid;
de1_psi=dpsi1-dpsid;


%control
es=0.01;
ke_phi_11=0.65;ke_phi_12=7/9;ke_phi_13=(2-ke_phi_12)*es^(ke_phi_12-1);ke_phi_14=(ke_phi_12-1)*es^(ke_phi_12-2);b1=0.65;
ke_theta_11=0.5;ke_theta_12=7/9;ke_theta_13=(2-ke_theta_12)*es^(ke_theta_12-1);ke_theta_14=(ke_theta_12-1)*es^(ke_theta_12-2);b2=0.5;
ke_psi_11=2.5;ke_psi_12=7/9;ke_psi_13=(2-ke_psi_12)*es^(ke_psi_12-1);ke_psi_14=(ke_psi_12-1)*es^(ke_psi_12-2);b3=2.5;


if abs(e1_phi)>es
    L_phi_1=ke_phi_11*((abs(e1_phi))^ke_phi_12)*sign(e1_phi);
else
    L_phi_1=ke_phi_13*e1_phi+ke_phi_14*e1_phi*e1_phi*sign(e1_phi);
end
if abs(e1_theta)>es
    L_theta_1=ke_theta_11*((abs(e1_theta))^ke_theta_12)*sign(e1_theta);
else
    L_theta_1=ke_theta_13*e1_theta+ke_theta_14*e1_theta*e1_theta*sign(e1_theta);
end
if abs(e1_psi)>es
    L_psi_1=ke_psi_11*((abs(e1_psi))^(ke_psi_12))*sign(e1_psi);
else
    L_psi_1=ke_psi_13*e1_psi+ke_psi_14*e1_psi*e1_psi*sign(e1_psi);
end
s_phi_1=de1_phi+b1*e1_phi+L_phi_1;
s_theta_1=de1_theta+b2*e1_theta+L_theta_1;
s_psi_1=de1_psi+b3*e1_psi+L_psi_1;

if abs(e1_phi)>es
    dL_phi_1=ke_phi_11*ke_phi_12*((abs(e1_phi))^(ke_phi_12-1))*de1_phi;
else 
    dL_phi_1=ke_phi_13*de1_phi+2*ke_phi_14*e1_phi*de1_phi*sign(e1_phi);
end
if abs(e1_theta)>es
    dL_theta_1=ke_theta_11*ke_theta_12*((abs(e1_theta))^(ke_theta_12-1))*de1_theta;
else
    dL_theta_1=ke_theta_13*de1_theta+2*ke_theta_14*e1_theta*de1_theta*sign(e1_theta);
end
if abs(e1_psi)>es
    dL_psi_1=ke_psi_11*ke_psi_12*((abs(e1_psi))^(ke_psi_12-1))*de1_psi;
else
    dL_psi_1=ke_psi_13*de1_psi+2*ke_psi_14*e1_psi*de1_psi*sign(e1_psi);
end

% 
tao_phi=Ix*(-d4_gu+(Iy-Iz)/Ix*dtheta1*dpsi1-K4*l/Ix*dphi1+ddphid-b1*de1_phi-dL_phi_1-5*s_phi_1-5*((abs(s_phi_1))^(5/7))*sign(s_phi_1));
tao_theta=Ix*(-d5_gu+(Iz-Ix)/Iy*dphi1*dpsi1-K5*l/Iy*dtheta1+ddthetad-b2*de1_theta-dL_theta_1-5*s_theta_1-5*((abs(s_theta_1))^(5/7))*sign(s_theta_1));
tao_psi=Ix*(-d6_gu+(Ix-Iy)/Iz*dphi1*dtheta1-K6/Iz*dpsi1+ddpsid-b3*de1_psi-dL_psi_1-5*s_psi_1-5*((abs(s_psi_1))^(5/7))*sign(s_psi_1));

== matlab function quav1/QUAV model1 ==
  data: dphi1 input double; dtheta1 input double; dpsi1 input double; Tao1 input double; Tao2 input double; Tao3 input double; ddphi1 output double; ddtheta1 output double; ddpsi1 output double; t input double; d4 output double; d5 output double; d6 output double
function [ddphi1,ddtheta1,ddpsi1,d4,d5,d6] = fcn(dphi1,dtheta1,dpsi1,Tao1,Tao2,Tao3,t)

%disturbance
d4=0.7*sin(t)+1.2*cos(2*t);
d5=0.5*sin(2*t)+1.5*cos(3*t);
d6=0.3*sin(3*t)+0.5*cos(2*t);

%parameter att
K4=0.1;K5=0.1;K6=0.1;
Ix=1.2416;Iy=1.2416;Iz=2.4832;l=0.2;

%
ddphi1=Tao1/Ix+dtheta1*dpsi1*(Iy-Iz)/Ix-l*K4*dphi1/Ix+d4;
ddtheta1=Tao2/Iy+dphi1*dpsi1*(Iz-Ix)/Iy-l*K5*dtheta1/Iy+d5;
ddpsi1=Tao3/Iz+dphi1*dtheta1*(Ix-Iy)/Iz-K6*dpsi1/Iz+d6;

== matlab function quav1/Disturbance Observer 2 ==
  data: dW_gu4 output double; dW_gu5 output double; dW_gu6 output double; dW_e_gu4 output double; dW_e_gu5 output double; dW_e_gu6 output double; dphi1 input double; dtheta1 input double; dpsi1 input double; Tao1 input double; Tao2 input double; Tao3 input double; W_gu4 input double; W_gu5 input double; W_gu6 input double; d4_gu output double; d5_gu output double; d6_gu output double; W_e_gu4 input double; W_e_gu5 input double; W_e_gu6 input double; dW_e4 input double; dW_e5 input double; dW_e6 input double; W_e4 output double; W_e5 output double; W_e6 output double

function [dW_gu4,dW_gu5,dW_gu6,dW_e_gu4,dW_e_gu5,dW_e_gu6,d4_gu,d5_gu,d6_gu,W_e4,W_e5,W_e6] = fcn(dphi1,dtheta1,dpsi1,Tao1,Tao2,Tao3,W_gu4,W_gu5,W_gu6,W_e_gu4,W_e_gu5,W_e_gu6,dW_e4,dW_e5,dW_e6)
m1=1;
m2=1;
m3=1;
m4=0.1;
m5=3/5;
m6=0.1;
m7=7/5;
m8=0.1;
K4=0.1;K5=0.1;K6=0.1;
Ix=1.2416;Iy=1.2416;Iz=2.4832;l=0.2;

W_e4=dphi1-W_gu4;
W_e5=dtheta1-W_gu5;
W_e6=dpsi1-W_gu6;

dW_gu4=Tao1/Ix+dtheta1*dpsi1*(Iy-Iz)/Ix-l*K4*dphi1/Ix+m1*W_e4;
dW_gu5=Tao2/Iy+dphi1*dpsi1*(Iz-Ix)/Iy-l*K5*dtheta1/Iy+m2*W_e5;
dW_gu6=Tao3/Iz+dphi1*dtheta1*(Ix-Iy)/Iz-K6*dpsi1/Iz+m3*W_e6;


W_e_e4=W_e_gu4-W_e4;
W_e_e5=W_e_gu5-W_e5;
W_e_e6=W_e_gu6-W_e6;

dW_e_gu4=dW_e4-m4*(sign(W_e_e4)*abs(W_e_e4)^m5)-m6*(sign(W_e_e4)*abs(W_e_e4)^m7)-m8*W_e_e4;
dW_e_gu5=dW_e5-m4*(sign(W_e_e5)*abs(W_e_e5)^m5)-m6*(sign(W_e_e5)*abs(W_e_e5)^m7)-m8*W_e_e5;
dW_e_gu6=dW_e6-m4*(sign(W_e_e6)*abs(W_e_e6)^m5)-m6*(sign(W_e_e6)*abs(W_e_e6)^m7)-m8*W_e_e6;


d4_gu=m1*W_e_gu4+dW_e4;
d5_gu=m2*W_e_gu5+dW_e5;
d6_gu=m3*W_e_gu6+dW_e6;

== matlab function MATLAB Function1 ==
  data: t input double; ox output double; oy output double; oz output double; vox output double; voy output double; voz output double; aox output double; aoy output double; aoz output double; r output double; is_dynamic output double
function [ox,oy,oz,vox,voy,voz,aox,aoy,aoz,r,is_dynamic] = fcn(t)
%% dynamic obstacle 1
% 
xc1 = 20;
yc1 = 19;
zc1 = 1;
% 
a = 4; b = 4; c = 4;
% 
T = 15;
omega = 2*pi / T;
% 
theta = omega * t;
phi = omega * t;
% 
ox1 = xc1 + a * cos(theta) * sin(phi);
oy1 = yc1 + b * sin(theta) * sin(phi);
oz1 = zc1 + c * cos(phi);
r1 = 4;  
% 
dtheta = omega;
dphi = omega;

vox1 = -a * sin(theta) * sin(phi) * dtheta + a * cos(theta) * cos(phi) * dphi;
voy1 =  b * cos(theta) * sin(phi) * dtheta + b * sin(theta) * cos(phi) * dphi;
voz1 = -c * sin(phi) * dphi;
% 
aox1 = -2 * a * omega^2 * (cos(theta)*sin(phi) + sin(theta)*cos(phi));
aoy1 = -2 * b * omega^2 * (sin(theta)*sin(phi) - cos(theta)*cos(phi));
aoz1 = -c * omega^2 * cos(phi);


%% dynamic obstacle 2
%
xc2 = 42; 
yc2 = 42; 
zc2 = 1; 
% 
a2 = 3; b2 = 3; c2 = 2; 
%  
T2 = 5; omega2 = 2*pi/T2; 
% 
theta2 = omega2 * t; 
% 
ox2 = xc2 + a2 * cos(theta2); 
oy2 = yc2 + b2 * sin(theta2); 
oz2 = zc2 + c2 * sin(theta2/2); 
% 
r2 = 3; 
% 
vox2 = -a2 * omega2 * sin(theta2);
voy2 =  b2 * omega2 * cos(theta2);
voz2 =  (c2 * omega2 / 2) * cos(theta2/2);
% 
aox2 = -a2 * omega2^2 * cos(theta2);
aoy2 = -b2 * omega2^2 * sin(theta2);
aoz2 = -(c2 * omega2^2 / 4) * sin(theta2/2);

%% dynamic obstacle 3
% 
xc6 = 47; 
yc6 = 47; 
zc6 = 1; 
% 
a6 = 2; b6 = 3; c6 = 2.5; 
%  
T6 = 8; omega6 = 2*pi/T6; 
% 
theta6 = omega6 * t; 
%  
ox6 = xc6 + a6 * cos(theta6); 
oy6 = yc6 + b6 * sin(theta6); 
oz6 = zc6 + c6 * sin(theta6/2); 
% 
r6 = 2; 
% 
vox6 = -a6 * omega6 * sin(theta6);
voy6 =  b6 * omega6 * cos(theta6);
voz6 =  (c6 * omega6 / 2) * cos(theta6/2);
% 
aox6 = -a6 * omega6^2 * cos(theta6);
aoy6 = -b6 * omega6^2 * sin(theta6);
aoz6 = -(c6 * omega6^2 / 4) * sin(theta6/2);

%% static obstacles

% static obstacle 1
ox3 = 10; oy3 = 9; oz3 = 1; r3 = 3;

% static obstacle 2
ox4 = 30; oy4 = 32; oz4 = 1; r4 = 3;

% static obstacle 3
ox5 = 38; oy5 = 34; oz5 = 1; r5 = 3;

%% All obstacles
% position 
ox = [ox1; ox2; ox3; ox4; ox5; ox6];
oy = [oy1; oy2; oy3; oy4; oy5; oy6];
oz = [oz1; oz2; oz3; oz4; oz5; oz6];

% 
r = [r1; r2; r3; r4; r5;r6];

% state
is_dynamic = [1; 1; 0; 0; 0; 1];

% speed
vox = [vox1; vox2; 0; 0; 0; vox6];
voy = [voy1; voy2; 0; 0 ;0; voy6];
voz = [voz1; voz2; 0; 0; 0; voz6];


% 
aox = [aox1; aox2; 0; 0; 0; aox6];
aoy = [aoy1; aoy2; 0; 0; 0; aoy6];
aoz = [aoz1; aoz2; 0; 0; 0; aoz6];









end
